simulink library "ExternalChimeProcessBtc"  (R2022b)
settings: Solver=VariableStepAuto  StartTime=0.0  StopTime=10.0  RelTol=1e-3
libraries: AnnVolumeBtc x1, HandyTextFile x1, RTC x1, ChimePoolDelayLibBtc x1, PoolIir x1, RouterBtc x1
settings Model: Creator=kl13806  LastModifiedBy=jz1055514
settings SolverCC: AlgebraicLoopSolver=TrustRegion
settings DebuggingCC: UnconnectedInputMsg=warning  UnconnectedOutputMsg=warning  UnconnectedLineMsg=warning  SFMachineParentedDataDiag=warning
settings ModelReferenceCC: EnableRefExpFcnMdlSchedulingChecks=on
settings RTWCC: DLArmComputeVersion=19.05

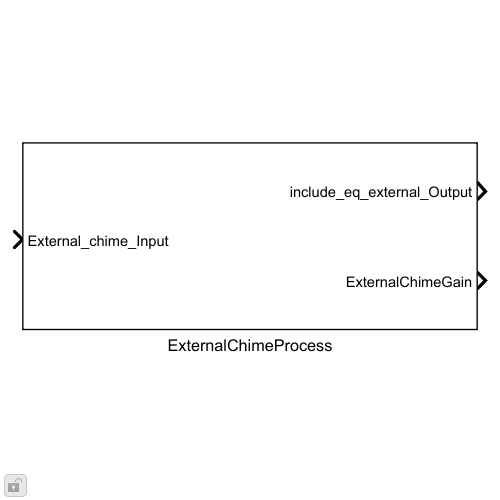
[thumbnail: Simulink's stored preview of the top-level diagram]
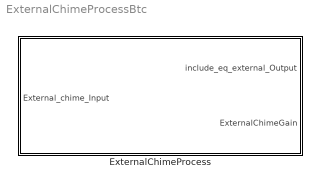
== system ExternalChimeProcessBtc ==
  ExternalChimeProcess : Subsystem  mask(Chimes ExternalChimeProcess){Config=[]}
      mask prompts: Config "ExternalChimeProcessConfig"
      mask init:
      | blkh=gcbh;
      | Config=BTConfig.Assert(blkh,Config);
      | 
      | Config.Validate();
      | 
      | %Flatten for MFBs
      | frameSize = Config.FrameSize;
      | numExtChimes = Config.NumExtChimes;

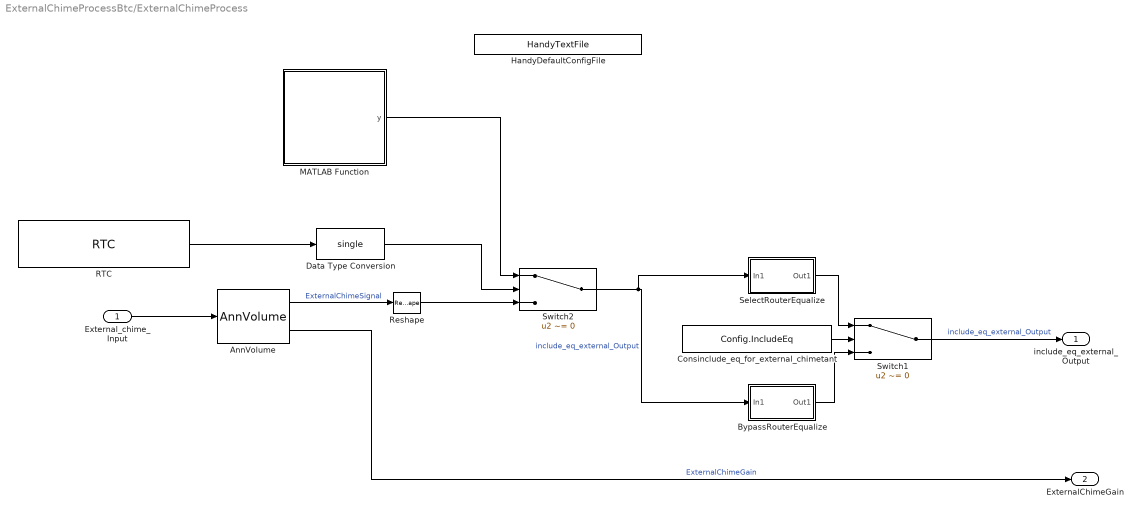
== system ExternalChimeProcessBtc/ExternalChimeProcess ==
  External_chime_Input : Inport
  AnnVolume : AnnVolumeBtc/AnnVolume  FeatureName=Volume  Config=Config.Volume  TriggerInit=[-40 195 40 255]
      settings: SourceProductName=Bose Blocklib
  BypassRouterEqualize : Subsystem  TreatAsAtomicUnit=on
  Consinclude_eq_for_external_chimetant : Constant  Value=Config.IncludeEq  VectorParams1D=off  OutDataTypeStr=boolean
  Data Type Conversion : DataTypeConversion  OutDataTypeStr=single  SaturateOnIntegerOverflow=off  RndMeth=Floor
  HandyDefaultConfigFile : HandyTextFile/HandyTextFile  TemplateSource=Config  FileSuffix=Init  OpenDialogOnLoad=off  UseThisBlockName=off  AddGrandParentNamePrefix=off  TheDefaultText=|  ShowInLibBrowser=on
      | % $(FILENAME) Setup model parameters for each "Init" callback (e.g. update diagram)
      | sample_rate_in_hertz = 44100;
      | frame_size = 32;
      | sysin_channel_count = 2;
      settings: SourceProductName=Bose Talaria
  MATLAB Function : MATLAB Function  TreatAsAtomicUnit=on
  RTC : RTC/RTC  REQ_Priority=RTC_Mask.NormalPriority  RequestAtInit=off  EnableRequest=off  REQElemName1=externalChimeCancel  REQElemType1=boolean  REQElemWidth1=length(Config.ExternalChimeCancel)  REQElemInitial1=Config.ExternalChimeCancel  REQElemType2=uint32  REQElemWidth2=1  REQElemInitial2=[]  REQElemType3=uint32  REQElemWidth3=1  REQElemInitial3=[]  REQElemType4=uint32  REQElemWidth4=1  REQElemInitial4=[]  REQElemType5=uint32  REQElemWidth5=1  REQElemInitial5=[]  REQElemType6=uint32  REQElemWidth6=1  REQElemInitial6=[]  REQElemType7=uint32  REQElemWidth7=1  REQElemInitial7=[]  REQElemType8=uint32  REQElemWidth8=1  REQElemInitial8=[]  REQElemType9=uint32  REQElemWidth9=1  REQElemInitial9=[]  REQElemType10=uint32  REQElemWidth10=1  REQElemInitial10=[]  EnableResponse=on  EnableRSP_StatusIn=off  RSPElemType1=boolean  RSPElemWidth1=1  RSPElemType2=uint32  RSPElemWidth2=1  RSPElemType3=uint32  RSPElemWidth3=1  RSPElemType4=uint32  RSPElemWidth4=1  RSPElemType5=uint32  RSPElemWidth5=1  RSPElemType6=uint32  RSPElemWidth6=1  RSPElemType7=uint32  RSPElemWidth7=1  RSPElemType8=uint32  RSPElemWidth8=1  RSPElemType9=uint32  RSPElemWidth9=1  RSPElemType10=uint32  RSPElemWidth10=1  EnableNotification=off  EnableNTF_PrepTrig=off  NTFElemType1=uint32  NTFElemWidth1=1  NTFElemType2=uint32  NTFElemWidth2=1  NTFElemType3=uint32  NTFElemWidth3=1  NTFElemType4=uint32  NTFElemWidth4=1  NTFElemType5=uint32  NTFElemWidth5=1  NTFElemType6=uint32  NTFElemWidth6=1  NTFElemType7=uint32  NTFElemWidth7=1  NTFElemType8=uint32  NTFElemWidth8=1  NTFElemType9=uint32  NTFElemWidth9=1  NTFElemType10=uint32  NTFElemWidth10=1  MaskMessageName=ExtChimeConfig
      settings: SourceProductName=Bose Talaria
  Reshape : Reshape  OutputDimensionality=Customize  OutputDimensions=[Config.FrameSize,Config.NumExtChimes]
  SelectRouterEqualize : Subsystem  TreatAsAtomicUnit=on
  Switch1 : Switch  Criteria=u2 ~= 0  SaturateOnIntegerOverflow=off  InputSameDT=off
  Switch2 : Switch  Criteria=u2 ~= 0  SaturateOnIntegerOverflow=off  InputSameDT=off
  include_eq_external_Output : Outport
  ExternalChimeGain : Outport  Port=2
  wires:
  BypassRouterEqualize/1(Out1) -> Switch1/3
  External_chime_Input/1 -> AnnVolume/1
  SelectRouterEqualize/1(Out1) -> Switch1/1
  Consinclude_eq_for_external_chimetant/1 -> Switch1/2
  Switch1/1 -> include_eq_external_Output/1  "include_eq_external_Output"
  AnnVolume/2 -> ExternalChimeGain/1  "ExternalChimeGain"
  AnnVolume/1 -> Reshape/1  "ExternalChimeSignal"
  RTC/1 -> Data Type Conversion/1
  Reshape/1 -> Switch2/3
  Switch2/1 -> BypassRouterEqualize/1(In1), SelectRouterEqualize/1(In1)  "include_eq_external_Output"
  Data Type Conversion/1 -> Switch2/2
  MATLAB Function/1(y) -> Switch2/1

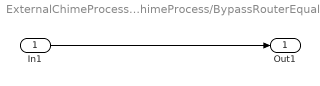
== system ExternalChimeProcessBtc/ExternalChimeProcess/BypassRouterEqualize ==
  In1 : Inport  OutDataTypeStr=single
  Out1 : Outport  OutDataTypeStr=single  VectorParamsAs1DForOutWhenUnconnected=off
  wires:
  In1/1 -> Out1/1

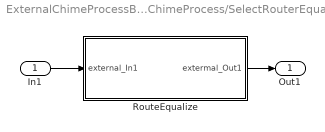
== system ExternalChimeProcessBtc/ExternalChimeProcess/SelectRouterEqualize ==
  In1 : Inport
  RouteEqualize : Subsystem
  Out1 : Outport  VectorParamsAs1DForOutWhenUnconnected=off
  wires:
  RouteEqualize/1(extermal_Out1) -> Out1/1
  In1/1 -> RouteEqualize/1(external_In1)

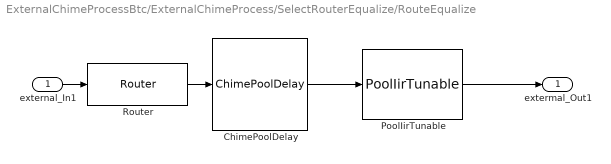
== system ExternalChimeProcessBtc/ExternalChimeProcess/SelectRouterEqualize/RouteEqualize ==
  external_In1 : Inport
  ChimePoolDelay : ChimePoolDelayLibBtc/ChimePoolDelay  Config=Config.PoolDelay  FeatureName=PoolDelay
      settings: SourceProductName=Bose Blocklib
  PoolIirTunable : PoolIir/PoolIirTunable  FeatureName=PoolIir  Config=Config.PoolIir
      settings: SourceProductName=Bose Blocklib
  Router : RouterBtc/Router  Config=Config.Router  FeatureName=Router
      settings: SourceProductName=Bose Blocklib
  extermal_Out1 : Outport  VectorParamsAs1DForOutWhenUnconnected=off
  wires:
  PoolIirTunable/1 -> extermal_Out1/1
  ChimePoolDelay/1 -> PoolIirTunable/1
  external_In1/1 -> Router/1
  Router/1 -> ChimePoolDelay/1

== matlab function ExternalChimeProcessBtc/ExternalChimeProcess/MATLAB Function ==
  data: y output size=[frameSize numExtChimes]; frameSize parameter size=[1 1]; numExtChimes parameter size=[1 1]
function y = fcn(frameSize, numExtChimes)
% simple function to pad zeros for the given frame size and number of
% channels
y = single(zeros(frameSize, numExtChimes));
